simulink model "and_or_combinational"  (R2018b)
settings: Solver=VariableStepAuto  StartTime=0.0  StopTime=30  RelTol=1e-3
settings Model: EnablePacing=on  Creator=kjartan  LastModifiedBy=kjartan

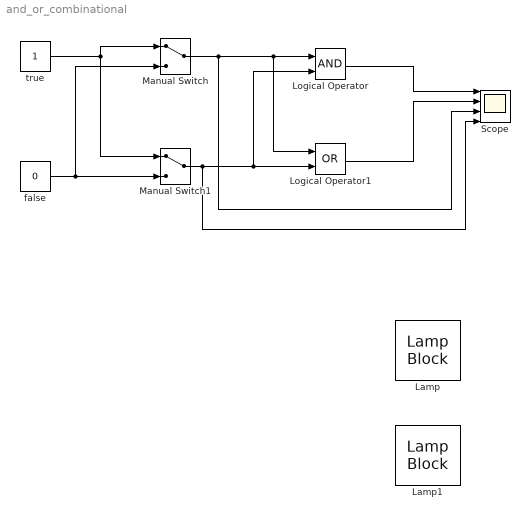
== system and_or_combinational ==
  Lamp : LampBlock  WebBlockId=9
  Lamp1 : LampBlock  WebBlockId=10
  Logical Operator : Logic  AllPortsSameDT=off  OutDataTypeStr=boolean
  Logical Operator1 : Logic  Operator=OR  AllPortsSameDT=off  OutDataTypeStr=boolean
  Manual Switch : ManualSwitch
  Manual Switch1 : ManualSwitch
  Scope : Scope  NumInputPorts=4
  false : Constant  Value=0
  true : Constant
  wires:
  true/1 -> Manual Switch1/1, Manual Switch/1
  false/1 -> Manual Switch1/2, Manual Switch/2
  Manual Switch/1 -> Scope/3, Logical Operator1/1, Logical Operator/1
  Manual Switch1/1 -> Scope/4, Logical Operator1/2, Logical Operator/2
  Logical Operator/1 -> Scope/1
  Logical Operator1/1 -> Scope/2
